simulink model "CONTROL_SYSTEM_V3_k"  (R2024a)
settings: Solver=ode1  StartTime=0.0  StopTime=inf  FixedStep=0.01  RelTol=1e-5
values from neighbouring files (symbols this model uses):
  Beta1 = 3*Omega_o    (= 15)    [CONTROL_SYSTEM_VAR.m]
  Beta2 = 3*(Omega_o^2)    (= 75)    [CONTROL_SYSTEM_VAR.m]
  Beta3 = (Omega_o^3)    (= 125)    [CONTROL_SYSTEM_VAR.m]
  Desire_Max = 255    [CONTROL_SYSTEM_VAR.m]
  Desire_Min = 0    [CONTROL_SYSTEM_VAR.m]
  Direction_Pin = 1    [CONTROL_SYSTEM_VAR.m]
  EN_Pin = 0    [CONTROL_SYSTEM_VAR.m]
  J_aet = 0.0035    [CONTROL_SYSTEM_VAR.m]
  Kd = 2    [CONTROL_SYSTEM_VAR.m]
  Ki = 4    [CONTROL_SYSTEM_VAR.m]
  Kn = 0.1    [CONTROL_SYSTEM_VAR.m]
  Kp = 1.4    [CONTROL_SYSTEM_VAR.m]
  omga_c = 10    [CONTROL_SYSTEM_VAR.m]
  roa = 0.24    [CONTROL_SYSTEM_VAR.m]
undefined symbols (not defined in the file or in its folder): sigbuilder_block
libraries: arduinolib x30, simulink_extras x14, simulink x5, slpidlib x4, spsOnDelayLib x2, slctrl_autotuning x2, slctrl_adaptive x1
(part 2 of 4)

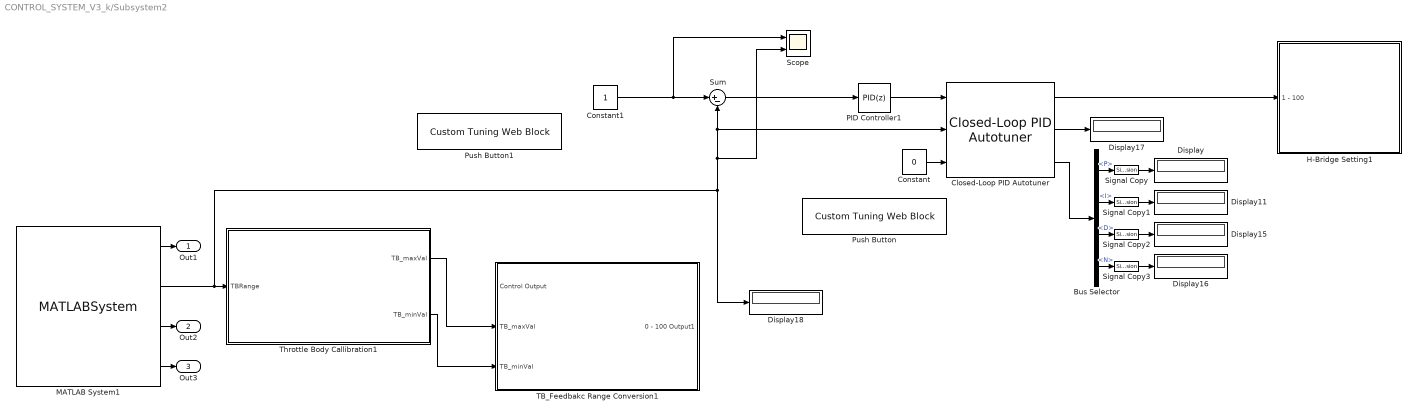
== system CONTROL_SYSTEM_V3_k/Subsystem2 ==
  Bus Selector : BusSelector  OutputSignals=P,I,D,N
  Closed-Loop PID Autotuner : slctrl_autotuning/Closed-Loop PID Autotuner  PIDType=PID  PIDForm=Parallel  TimeDomain=discrete-time  DiscreteTs=0.1  TuningTs=0.2  UseTuningTs=off  IntegratorFormula=Forward Euler  FilterFormula=Forward Euler  ContinuousTs=-1  Bandwidth=1  UseExternalWC=off  TargetPM=60  UseExternalPM=off  UseExternalAchievedPM=off  ExperimentMode=Superposition  PlantType=Stable  PlantSign=Positive  AmpSine=1  UseExternalAmpSine=off  UseExternalFRD=off  UseExternalU0=off  UseCompanion=off  NotDeployTuningModule=off  UsePLCCoder=off  OutputMode=control action + perturbation  BlockDataType=double  UseConnectedPID=on  blockpath=[]  tunedP=0  tunedI=0  tunedD=0  tunedN=100  tunedPM=0  EstimationWindowSize=3  UseExternalTuningParams=off  SingleMultiRateVariant=SingleSamplingRate  NumEstimationPeriods=4  NumSettlingPeriods=2  NumOfPRBSPeriod=1  PRBSSignalOrder=12  ExperimentModeVariant=VariantSuperimposed  OutputChoice=VariantCandD
      settings: LibrarySourceBlock=slctrlblks/Autotuning/Closed-Loop PID Autotuner
  Constant : Constant  Value=0
  Constant1 : Constant
  Display{,11,15..18} (6 alike) : Display
  H-Bridge Setting1 : Subsystem
      mask Display: image('H-Bridge.JPG');
  MATLAB System1 : MATLABSystem  System=ADS1115_Vread  SetGain=int16( 16 )  SampleTime=-1
      mask Type: ADS1115_Vread
      mask Display:
      | color('white');plot([100,100,100,100]*1,[100,100,100,100]*1);plot([100,100,100,100]*0,[100,100,100,100]*0);color('blue');text(38, 92, 'IO Device Builder','horizontalAlignment', 'right');
      | color('black');text(52,50,' ADS1115_Vread','horizontalAlignment','center');
      | port_label('output',1,'V0');port_label('output',2,'V1');port_label('output',3,'V2');port_label('output',4,'V3');
  PID Controller1 : slpidlib/PID Controller  Controller=PID  Form=Parallel  TimeDomain=Discrete-time  UseExternalTs=off  SampleTime=-1  IntegratorMethod=Forward Euler  FilterMethod=Forward Euler  ControllerParametersSource=internal  P=0  I=185.8371  UseKiTs=off  D=87.2762  UseExternalDerivativeSource=off  N=100  UseFilter=on  TunerSelectOption=Transfer Function Based (PID Tuner App)  InitialConditionSource=internal  InitialConditionForIntegrator=0  InitialConditionForFilter=0  DifferentiatorICPrevScaledInput=0  ExternalReset=none  TrackingMode=off  Kt=1  LimitOutput=off  SatLimitsSource=internal  UpperSaturationLimit=inf  LowerSaturationLimit=-inf  LinearizeAsGain=on  AntiWindupMode=none  Kb=1  LimitIntegrator=off  UpperIntegratorSaturationLimit=inf  LowerIntegratorSaturationLimit=-inf  POutMin=[]  POutMax=[]  IOutMin=[]  IOutMax=[]  DOutMin=[]  DOutMax=[]  NOutMin=[]  NOutMax=[]  SumOutMin=[]  SumOutMax=[]  SaturationOutMin=[]  SaturationOutMax=[]  PParamMin=[]  PParamMax=[]  IParamMin=[]  IParamMax=[]  DParamMin=[]  DParamMax=[]  NParamMin=[]  NParamMax=[]  KbParamMin=[]  KbParamMax=[]  KtParamMin=[]  KtParamMax=[]  KbOutMin=[]  KbOutMax=[]  KtOutMin=[]  KtOutMax=[]  IntegratorOutMin=[]  IntegratorOutMax=[]  FilterOutMin=[]  FilterOutMax=[]  SumI1OutMin=[]  SumI1OutMax=[]  SumI2OutMin=[]  SumI2OutMax=[]  SumI3OutMin=[]  SumI3OutMax=[]  SumI4OutMin=[]  SumI4OutMax=[]  SumDOutMin=[]  SumDOutMax=[]  DifferentiatorOutMin=[]  DifferentiatorOutMax=[]  FilterDiffOutCoefMin=[]  FilterDiffOutCoefMax=[]  ReciprocalOutMin=[]  ReciprocalOutMax=[]  SumDenOutMin=[]  SumDenOutMax=[]  SumNumOutMin=[]  SumNumOutMax=[]  DivideOutMin=[]  DivideOutMax=[]  UdiffTsProdOutMin=[]  UdiffTsProdOutMax=[]  NTsProdOutMin=[]  NTsProdOutMax=[]  UintegralTsProdOutMin=[]  UintegralTsProdOutMax=[]  UngainTsProdOutMin=[]  UngainTsProdOutMax=[]  ClampingZeroOutDataTypeStr=Inherit: Inherit via back propagation  ClampingZeroOutMin=[]  ClampingZeroOutMax=[]  FilterDenConstantOutDataTypeStr=Inherit: Inherit via back propagation  FilterDenConstantOutMin=[]  FilterDenConstantOutMax=[]  PCopyOutDataTypeStr=Inherit: Inherit via back propagation  PCopyOutMin=[]  PCopyOutMax=[]  NCopyOutDataTypeStr=Inherit: Inherit via back propagation  NCopyOutMin=[]  NCopyOutMax=[]  IntegratorContinuousStateAttributes=''  IntegratorStateMustResolveToSignalObject=off  IntegratorRTWStateStorageClass=Auto  FilterContinuousStateAttributes=''  FilterStateMustResolveToSignalObject=off  FilterRTWStateStorageClass=Auto  ParallelPVariant=InternalParameters  IdealPVariant=Disabled  IVariant=InternalParameters  DVariant=InternalParameters  IntegratorVariant=Discrete  SatVariant=Disabled  AWVariant=Passthrough  PCopyVariant=Disabled  TRVariant=Disabled  FdbkBlocksVariant=Forward  IdealPFdbkVariant=Disabled  SatFdbkVariant=Disabled  DerivativeFilterVariant=ForwardEulerFilter  NVariant=InternalParameters  NCopyVariant=Disabled  FilterICVariant=InternalICsFilter  IntegratorICVariant=InternalICs  ExternalResetVariant=Disabled  TRSumVariant=Passthrough  SumFdbkVariant=Disabled  SumVariant=Sum_PID  TsampFilterVariant=InternalTs  TsampNgainVariant=Passthrough  TsampIntegralVariant=Disabled_SignalSpec  ExternalSaturationOutDataTypeStr=Inherit: Same as second input  DerivativeSourceVariant=ErrorSignal
  Push Button : CustomTuningWebBlock  LabelPosition=Hide  ShowInitialText=on  Configuration="{\"components\":[{\"name\":\"BackgroundImageComponent\",\"settings\":{\"image\":{\"size\":[0,0],\"src\":\"default\",\"srcOrientation\":\"horizontal\"},\"position\":[0,0,1,1],\"scaleMode\":\"0\"}},{\"name\":\"ButtonStateComponent\",\"settings\":{\"buttonType\":\"latch\",\"clickFcn\":\"\",\"image\":{\"size\":[180,45],\"srcOrientation\":\"Right\"},\"latched\":false,\"offValue\":null,\"onValue\":\"1\",\"position\":[0,0,1,1],\"pressDelay\":\"500\",\"pressFcn\":\"\",\"repeatInterval\":\"0\",\"states\":[{\"horizontalAlignment\":\"center\",\"image\":{\"position\":[0.04444444444444445,0.005555555555555536,0.9888888888888889,0.9111111111111111],\"size\":[0.9888888888888889,0.9111111111111111],\"src\":\"data:image\\/svg+xml;base64,PHN2ZyB4bWxucz0iaHR0cDovL3d3dy53My5vcmcvMjAwMC9zdmciIHhtbG5zOnhsaW5rPSJodHRwOi8vd3d3LnczLm9yZy8xOTk5L3hsaW5rIiB2aWV3Qm94PSIwIDAgMTc3LjI1IDQwLjg4Ij48ZGVmcz48c3R5bGU+LmNscy0xe2ZpbGw6dXJsKCNyYWRpYWwtZ3JhZGllbnQpO30uY2xzLTJ7ZmlsbDp1cmwoI2xpbmVhci1ncmFkaWVudCk7fS5jbHMtM3tmaWxsOnVybCgjbGluZWFyLWdyYWRpZW50LTIpO308L3N0eWxlPjxyYWRpYWxHcmFkaWVudCBpZD0icmFkaWFsLWdyYWRpZW50IiBjeD0iOTAuMDkiIGN5PSIyMi42NiIgcj0i ...(+2212 chars)\",\"srcOrientation\":\"Right\"},\"label\":{\"color\":[1,1,0.78,1],\"icon\":{\"size\":[0.1,0.375],\"src\":\"data:image\\/svg+xml;base64,PHN2ZyBpZD0iT2ZmIiB4bWxucz0iaHR0cDovL3d3dy53My5vcmcvMjAwMC9zdmciIHhtbG5zOnhsaW5rPSJodHRwOi8vd3d3LnczLm9yZy8xOTk5L3hsaW5rIiB2aWV3Qm94PSIwIDAgNTAgNTAiPjxkZWZzPjxzdHlsZT4uY2xzLTF7ZmlsbDojN2Y4MDgwO3N0cm9rZTojMjcyNjI2O3N0cm9rZS1taXRlcmxpbWl0OjEwO3N0cm9rZS13aWR0aDozcHg7fS5jbHMtMntmaWxsOnVybCgjbGluZWFyLWdyYWRpZW50KTt9PC9zdHlsZT48bGluZWFyR3JhZGllbnQgaWQ9ImxpbmVhci1ncmFkaWVudCIgeDE9IjI1IiB5MT0iOSIgeDI9IjI1IiB5Mj0iMzciIGdyYWRpZW50VW5pdHM9InVzZXJTcGFjZU9uVXNlIj48c3RvcCBvZmZzZXQ9IjAiIHN0b3AtY29sb3I9IiNmZmYiIHN0b3Atb3BhY2l0eT0iMC43NSIvPjxzdG9wIG9mZnNldD0iMSIgc3RvcC1jb2xvcj0iI2ZmZiIgc3RvcC1vcGFjaXR5PSIwIi8+PC9saW5lYXJHcmFkaWVudD48L2RlZnM+PGNpcmNsZSBjbGFzcz0iY2xzLTEiIGN4PSIyNSIgY3k9IjI1IiByPSIyMCIvPjxjaXJjbGUgY2xhc3M9ImNscy0yIiBjeD0iMjUiIGN5PSIyMyIgcj0iMTQiLz48L3N2Zz4=\",\"srcOrientation\":\"Right\"},\"iconPlacement\":\"left\",\"opacity\":1,\"show\":true,\"text\":{\"content\":\"Button\",\"font\":\"Helvetica\",\"fontSize\":14}},\"labelOffset\":[0,0],\"verticalAlignment\":\"middle\"},{\"horizontalAlignment\":\"center\",\"image\":{\"position\":[0.04444444444444445,0.005555555555555536,0.9888888888888889,0.9111111111111111],\"size\":[0.9888888888888889,0.9111111111111111],\"src\":\"data:image\\/svg+xml;base64,PHN2ZyB4bWxucz0iaHR0cDovL3d3dy53My5vcmcvMjAwMC9zdmciIHhtbG5zOnhsaW5rPSJodHRwOi8vd3d3LnczLm9yZy8xOTk5L3hsaW5rIiB2aWV3Qm94PSIwIDAgMTc3LjI1IDQwLjg4Ij48ZGVmcz48c3R5bGU+LmNscy0xe2ZpbGw6dXJsKCNyYWRpYWwtZ3JhZGllbnQpO30uY2xzLTJ7ZmlsbDp1cmwoI2xpbmVhci1ncmFkaWVudCk7fS5jbHMtM3tmaWxsOnVybCgjbGluZWFyLWdyYWRpZW50LTIpO308L3N0eWxlPjxyYWRpYWxHcmFkaWVudCBpZD0icmFkaWFsLWdyYWRpZW50IiBjeD0iOTAuMDkiIGN5PSIyMi42NiIgcj0i ...(+2216 chars)\",\"srcOrientation\":\"Right\"},\"label\":{\"color\":[1,1,0.78,1],\"icon\":{\"size\":[0.1,0.375],\"src\":\"data:image\\/svg+xml;base64,PHN2ZyB4bWxucz0iaHR0cDovL3d3dy53My5vcmcvMjAwMC9zdmciIHhtbG5zOnhsaW5rPSJodHRwOi8vd3d3LnczLm9yZy8xOTk5L3hsaW5rIiB2aWV3Qm94PSIwIDAgNTAgNTAiPjxkZWZzPjxzdHlsZT4uY2xzLTF7ZmlsbDojNmFiZDQ1O3N0cm9rZTojMjcyNjI2O3N0cm9rZS1taXRlcmxpbWl0OjEwO3N0cm9rZS13aWR0aDozcHg7fS5jbHMtMntmaWxsOnVybCgjbGluZWFyLWdyYWRpZW50KTt9PC9zdHlsZT48bGluZWFyR3JhZGllbnQgaWQ9ImxpbmVhci1ncmFkaWVudCIgeDE9IjI1IiB5MT0iOSIgeDI9IjI1IiB5Mj0iMzciIGdyYWRpZW50VW5pdHM9InVzZXJTcGFjZU9uVXNlIj48c3RvcCBvZmZzZXQ9IjAiIHN0b3AtY29sb3I9IiNmZmYiIHN0b3Atb3BhY2l0eT0iMC43NSIvPjxzdG9wIG9mZnNldD0iMSIgc3RvcC1jb2xvcj0iI2ZmZiIgc3RvcC1vcGFjaXR5PSIwIi8+PC9saW5lYXJHcmFkaWVudD48L2RlZnM+PGcgaWQ9Ik9uIj48Y2lyY2xlIGNsYXNzPSJjbHMtMSIgY3g9IjI1IiBjeT0iMjUiIHI9IjIwIi8+PGNpcmNsZSBjbGFzcz0iY2xzLTIiIGN4PSIyNSIgY3k9IjIzIiByPSIxNCIvPjwvZz48L3N2Zz4=\",\"srcOrientation\":\"Right\"},\"iconPlacement\":\"left\",\"opacity\":1,\"show\":true,\"text\":{\"content\":\"Button\",\"font\":\"Helvetica\",\"fontSize\":14}},\"labelOffset\":[0.025,0],\"verticalAlignment\":\"middle\"},{\"horizontalAlignment\":\"center\",\"image\":{\"position\":[0.04444444444444445,0.005555555555555536,0.9888888888888889,0.9111111111111111],\"size\":[0.9888888888888889,0.9111111111111111],\"src\":\"data:image\\/svg+xml;base64,PHN2ZyB4bWxucz0iaHR0cDovL3d3dy53My5vcmcvMjAwMC9zdmciIHhtbG5zOnhsaW5rPSJodHRwOi8vd3d3LnczLm9yZy8xOTk5L3hsaW5rIiB2aWV3Qm94PSIwIDAgMTc3LjI1IDQwLjg4Ij48ZGVmcz48c3R5bGU+LmNscy0xe2ZpbGw6dXJsKCNyYWRpYWwtZ3JhZGllbnQpO30uY2xzLTJ7ZmlsbDp1cmwoI2xpbmVhci1ncmFkaWVudCk7fS5jbHMtM3tmaWxsOnVybCgjbGluZWFyLWdyYWRpZW50LTIpO308L3N0eWxlPjxyYWRpYWxHcmFkaWVudCBpZD0icmFkaWFsLWdyYWRpZW50IiBjeD0iOTAuMDkiIGN5PSIyMi42NiIgcj0i ...(+2212 chars)\",\"srcOrientation\":\"Right\"},\"label\":{\"color\":[1,1,0.78,1],\"icon\":{\"size\":[0.1,0.375],\"src\":\"data:image\\/svg+xml;base64,PHN2ZyB4bWxucz0iaHR0cDovL3d3dy53My5vcmcvMjAwMC9zdmciIHhtbG5zOnhsaW5rPSJodHRwOi8vd3d3LnczLm9yZy8xOTk5L3hsaW5rIiB2aWV3Qm94PSIwIDAgNTAgNTAiPjxkZWZzPjxzdHlsZT4uY2xzLTF7ZmlsbDojNmFiZDQ1O3N0cm9rZTojMjcyNjI2O3N0cm9rZS1taXRlcmxpbWl0OjEwO3N0cm9rZS13aWR0aDozcHg7fS5jbHMtMntmaWxsOnVybCgjbGluZWFyLWdyYWRpZW50KTt9PC9zdHlsZT48bGluZWFyR3JhZGllbnQgaWQ9ImxpbmVhci1ncmFkaWVudCIgeDE9IjI1IiB5MT0iOSIgeDI9IjI1IiB5Mj0iMzciIGdyYWRpZW50VW5pdHM9InVzZXJTcGFjZU9uVXNlIj48c3RvcCBvZmZzZXQ9IjAiIHN0b3AtY29sb3I9IiNmZmYiIHN0b3Atb3BhY2l0eT0iMC43NSIvPjxzdG9wIG9mZnNldD0iMSIgc3RvcC1jb2xvcj0iI2ZmZiIgc3RvcC1vcGFjaXR5PSIwIi8+PC9saW5lYXJHcmFkaWVudD48L2RlZnM+PGcgaWQ9Ik9uIj48Y2lyY2xlIGNsYXNzPSJjbHMtMSIgY3g9IjI1IiBjeT0iMjUiIHI9IjIwIi8+PGNpcmNsZSBjbGFzcz0iY2xzLTIiIGN4PSIyNSIgY3k9IjIzIiByPSIxNCIvPjwvZz48L3N2Zz4=\",\"srcOrientation\":\"Right\"},\"iconPlacement\":\"left\",\"opacity\":1,\"show\":true,\"text\":{\"content\":\"Button\",\"font\":\"Helvetica\",\"fontSize\":14}},\"labelOffset\":[0,0],\"verticalAlignment\":\"middle\"},{\"horizontalAlignment\":\"center\",\"image\":{\"position\":[0.04444444444444445,0.005555555555555536,0.9888888888888889,0.9111111111111111],\"size\":[0.9888888888888889,0.9111111111111111],\"src\":\"data:image\\/svg+xml;base64,PHN2ZyB4bWxucz0iaHR0cDovL3d3dy53My5vcmcvMjAwMC9zdmciIHhtbG5zOnhsaW5rPSJodHRwOi8vd3d3LnczLm9yZy8xOTk5L3hsaW5rIiB2aWV3Qm94PSIwIDAgMTc3LjI1IDQwLjg4Ij48ZGVmcz48c3R5bGU+LmNscy0xe2ZpbGw6dXJsKCNyYWRpYWwtZ3JhZGllbnQpO30uY2xzLTJ7ZmlsbDp1cmwoI2xpbmVhci1ncmFkaWVudCk7fS5jbHMtM3tmaWxsOnVybCgjbGluZWFyLWdyYWRpZW50LTIpO308L3N0eWxlPjxyYWRpYWxHcmFkaWVudCBpZD0icmFkaWFsLWdyYWRpZW50IiBjeD0iOTAuMDkiIGN5PSIyMi42NiIgcj0i ...(+2216 chars)\",\"srcOrientation\":\"Right\"},\"label\":{\"color\":[1,1,0.78,1],\"icon\":{\"size\":[0.1,0.375],\"src\":\"data:image\\/svg+xml;base64,PHN2ZyBpZD0iT2ZmIiB4bWxucz0iaHR0cDovL3d3dy53My5vcmcvMjAwMC9zdmciIHhtbG5zOnhsaW5rPSJodHRwOi8vd3d3LnczLm9yZy8xOTk5L3hsaW5rIiB2aWV3Qm94PSIwIDAgNTAgNTAiPjxkZWZzPjxzdHlsZT4uY2xzLTF7ZmlsbDojN2Y4MDgwO3N0cm9rZTojMjcyNjI2O3N0cm9rZS1taXRlcmxpbWl0OjEwO3N0cm9rZS13aWR0aDozcHg7fS5jbHMtMntmaWxsOnVybCgjbGluZWFyLWdyYWRpZW50KTt9PC9zdHlsZT48bGluZWFyR3JhZGllbnQgaWQ9ImxpbmVhci1ncmFkaWVudCIgeDE9IjI1IiB5MT0iOSIgeDI9IjI1IiB5Mj0iMzciIGdyYWRpZW50VW5pdHM9InVzZXJTcGFjZU9uVXNlIj48c3RvcCBvZmZzZXQ9IjAiIHN0b3AtY29sb3I9IiNmZmYiIHN0b3Atb3BhY2l0eT0iMC43NSIvPjxzdG9wIG9mZnNldD0iMSIgc3RvcC1jb2xvcj0iI2ZmZiIgc3RvcC1vcGFjaXR5PSIwIi8+PC9saW5lYXJHcmFkaWVudD48L2RlZnM+PGNpcmNsZSBjbGFzcz0iY2xzLTEiIGN4PSIyNSIgY3k9IjI1IiByPSIyMCIvPjxjaXJjbGUgY2xhc3M9ImNscy0yIiBjeD0iMjUiIGN5PSIyMyIgcj0iMTQiLz48L3N2Zz4=\",\"srcOrientation\":\"Right\"},\"iconPlacement\":\"left\",\"opacity\":1,\"show\":true,\"text\":{\"content\":\"Button\",\"font\":\"Helvetica\",\"fontSize\":14}},\"labelOffset\":[0.025,0],\"verticalAlignment\":\"middle\"}]}},{\"name\":\"ForegroundImageComponent\",\"settings\":{\"image\":{\"size\":[0,0],\"src\":\"default\",\"srcOrientation\":\"horizontal\"},\"isForeground\":1,\"position\":[0,0,1,1],\"scaleMode\":\"0\"}}],\"settings\":{\"BindingType\":\"param\",\"aspectRatio\":3.7777777777777777,\"backgroundColor\":[0,0,0,\"1\"],\"backgroundOffset\":0,\"backgroundOpacity\":1,\"fixedAspectRatio\":\"on\",\"foregroundColor\":[252,252,196],\"showBackgroundColor\":false,\"variant\":\"push\",\"version\":\"R2023a\"},\"type\":\"Button\"}"
  Push Button1 : CustomTuningWebBlock  LabelPosition=Hide  ShowInitialText=on  Configuration="{\"components\":[{\"name\":\"BackgroundImageComponent\",\"settings\":{\"image\":{\"size\":[0,0],\"src\":\"default\",\"srcOrientation\":\"horizontal\"},\"position\":[0,0,1,1],\"scaleMode\":\"0\"}},{\"name\":\"ButtonStateComponent\",\"settings\":{\"buttonType\":\"latch\",\"clickFcn\":\"\",\"image\":{\"size\":[180,45],\"srcOrientation\":\"Right\"},\"latched\":true,\"offValue\":0,\"onValue\":\"1\",\"position\":[0,0,1,1],\"pressDelay\":\"500\",\"pressFcn\":\"\",\"repeatInterval\":\"0\",\"states\":[{\"horizontalAlignment\":\"center\",\"image\":{\"position\":[0.04444444444444445,0.005555555555555536,0.9888888888888889,0.9111111111111111],\"size\":[0.9888888888888889,0.9111111111111111],\"src\":\"data:image\\/svg+xml;base64,PHN2ZyB4bWxucz0iaHR0cDovL3d3dy53My5vcmcvMjAwMC9zdmciIHhtbG5zOnhsaW5rPSJodHRwOi8vd3d3LnczLm9yZy8xOTk5L3hsaW5rIiB2aWV3Qm94PSIwIDAgMTc3LjI1IDQwLjg4Ij48ZGVmcz48c3R5bGU+LmNscy0xe2ZpbGw6dXJsKCNyYWRpYWwtZ3JhZGllbnQpO30uY2xzLTJ7ZmlsbDp1cmwoI2xpbmVhci1ncmFkaWVudCk7fS5jbHMtM3tmaWxsOnVybCgjbGluZWFyLWdyYWRpZW50LTIpO308L3N0eWxlPjxyYWRpYWxHcmFkaWVudCBpZD0icmFkaWFsLWdyYWRpZW50IiBjeD0iOTAuMDkiIGN5PSIyMi42NiIgcj0i ...(+2212 chars)\",\"srcOrientation\":\"Right\"},\"label\":{\"color\":[1,1,0.78,1],\"icon\":{\"size\":[0.1,0.375],\"src\":\"data:image\\/svg+xml;base64,PHN2ZyBpZD0iT2ZmIiB4bWxucz0iaHR0cDovL3d3dy53My5vcmcvMjAwMC9zdmciIHhtbG5zOnhsaW5rPSJodHRwOi8vd3d3LnczLm9yZy8xOTk5L3hsaW5rIiB2aWV3Qm94PSIwIDAgNTAgNTAiPjxkZWZzPjxzdHlsZT4uY2xzLTF7ZmlsbDojN2Y4MDgwO3N0cm9rZTojMjcyNjI2O3N0cm9rZS1taXRlcmxpbWl0OjEwO3N0cm9rZS13aWR0aDozcHg7fS5jbHMtMntmaWxsOnVybCgjbGluZWFyLWdyYWRpZW50KTt9PC9zdHlsZT48bGluZWFyR3JhZGllbnQgaWQ9ImxpbmVhci1ncmFkaWVudCIgeDE9IjI1IiB5MT0iOSIgeDI9IjI1IiB5Mj0iMzciIGdyYWRpZW50VW5pdHM9InVzZXJTcGFjZU9uVXNlIj48c3RvcCBvZmZzZXQ9IjAiIHN0b3AtY29sb3I9IiNmZmYiIHN0b3Atb3BhY2l0eT0iMC43NSIvPjxzdG9wIG9mZnNldD0iMSIgc3RvcC1jb2xvcj0iI2ZmZiIgc3RvcC1vcGFjaXR5PSIwIi8+PC9saW5lYXJHcmFkaWVudD48L2RlZnM+PGNpcmNsZSBjbGFzcz0iY2xzLTEiIGN4PSIyNSIgY3k9IjI1IiByPSIyMCIvPjxjaXJjbGUgY2xhc3M9ImNscy0yIiBjeD0iMjUiIGN5PSIyMyIgcj0iMTQiLz48L3N2Zz4=\",\"srcOrientation\":\"Right\"},\"iconPlacement\":\"left\",\"opacity\":1,\"show\":true,\"text\":{\"content\":\"Button\",\"font\":\"Helvetica\",\"fontSize\":14}},\"labelOffset\":[0,0],\"verticalAlignment\":\"middle\"},{\"horizontalAlignment\":\"center\",\"image\":{\"position\":[0.04444444444444445,0.005555555555555536,0.9888888888888889,0.9111111111111111],\"size\":[0.9888888888888889,0.9111111111111111],\"src\":\"data:image\\/svg+xml;base64,PHN2ZyB4bWxucz0iaHR0cDovL3d3dy53My5vcmcvMjAwMC9zdmciIHhtbG5zOnhsaW5rPSJodHRwOi8vd3d3LnczLm9yZy8xOTk5L3hsaW5rIiB2aWV3Qm94PSIwIDAgMTc3LjI1IDQwLjg4Ij48ZGVmcz48c3R5bGU+LmNscy0xe2ZpbGw6dXJsKCNyYWRpYWwtZ3JhZGllbnQpO30uY2xzLTJ7ZmlsbDp1cmwoI2xpbmVhci1ncmFkaWVudCk7fS5jbHMtM3tmaWxsOnVybCgjbGluZWFyLWdyYWRpZW50LTIpO308L3N0eWxlPjxyYWRpYWxHcmFkaWVudCBpZD0icmFkaWFsLWdyYWRpZW50IiBjeD0iOTAuMDkiIGN5PSIyMi42NiIgcj0i ...(+2216 chars)\",\"srcOrientation\":\"Right\"},\"label\":{\"color\":[1,1,0.78,1],\"icon\":{\"size\":[0.1,0.375],\"src\":\"data:image\\/svg+xml;base64,PHN2ZyB4bWxucz0iaHR0cDovL3d3dy53My5vcmcvMjAwMC9zdmciIHhtbG5zOnhsaW5rPSJodHRwOi8vd3d3LnczLm9yZy8xOTk5L3hsaW5rIiB2aWV3Qm94PSIwIDAgNTAgNTAiPjxkZWZzPjxzdHlsZT4uY2xzLTF7ZmlsbDojNmFiZDQ1O3N0cm9rZTojMjcyNjI2O3N0cm9rZS1taXRlcmxpbWl0OjEwO3N0cm9rZS13aWR0aDozcHg7fS5jbHMtMntmaWxsOnVybCgjbGluZWFyLWdyYWRpZW50KTt9PC9zdHlsZT48bGluZWFyR3JhZGllbnQgaWQ9ImxpbmVhci1ncmFkaWVudCIgeDE9IjI1IiB5MT0iOSIgeDI9IjI1IiB5Mj0iMzciIGdyYWRpZW50VW5pdHM9InVzZXJTcGFjZU9uVXNlIj48c3RvcCBvZmZzZXQ9IjAiIHN0b3AtY29sb3I9IiNmZmYiIHN0b3Atb3BhY2l0eT0iMC43NSIvPjxzdG9wIG9mZnNldD0iMSIgc3RvcC1jb2xvcj0iI2ZmZiIgc3RvcC1vcGFjaXR5PSIwIi8+PC9saW5lYXJHcmFkaWVudD48L2RlZnM+PGcgaWQ9Ik9uIj48Y2lyY2xlIGNsYXNzPSJjbHMtMSIgY3g9IjI1IiBjeT0iMjUiIHI9IjIwIi8+PGNpcmNsZSBjbGFzcz0iY2xzLTIiIGN4PSIyNSIgY3k9IjIzIiByPSIxNCIvPjwvZz48L3N2Zz4=\",\"srcOrientation\":\"Right\"},\"iconPlacement\":\"left\",\"opacity\":1,\"show\":true,\"text\":{\"content\":\"Button\",\"font\":\"Helvetica\",\"fontSize\":14}},\"labelOffset\":[0.025,0],\"verticalAlignment\":\"middle\"},{\"horizontalAlignment\":\"center\",\"image\":{\"position\":[0.04444444444444445,0.005555555555555536,0.9888888888888889,0.9111111111111111],\"size\":[0.9888888888888889,0.9111111111111111],\"src\":\"data:image\\/svg+xml;base64,PHN2ZyB4bWxucz0iaHR0cDovL3d3dy53My5vcmcvMjAwMC9zdmciIHhtbG5zOnhsaW5rPSJodHRwOi8vd3d3LnczLm9yZy8xOTk5L3hsaW5rIiB2aWV3Qm94PSIwIDAgMTc3LjI1IDQwLjg4Ij48ZGVmcz48c3R5bGU+LmNscy0xe2ZpbGw6dXJsKCNyYWRpYWwtZ3JhZGllbnQpO30uY2xzLTJ7ZmlsbDp1cmwoI2xpbmVhci1ncmFkaWVudCk7fS5jbHMtM3tmaWxsOnVybCgjbGluZWFyLWdyYWRpZW50LTIpO308L3N0eWxlPjxyYWRpYWxHcmFkaWVudCBpZD0icmFkaWFsLWdyYWRpZW50IiBjeD0iOTAuMDkiIGN5PSIyMi42NiIgcj0i ...(+2212 chars)\",\"srcOrientation\":\"Right\"},\"label\":{\"color\":[1,1,0.78,1],\"icon\":{\"size\":[0.1,0.375],\"src\":\"data:image\\/svg+xml;base64,PHN2ZyB4bWxucz0iaHR0cDovL3d3dy53My5vcmcvMjAwMC9zdmciIHhtbG5zOnhsaW5rPSJodHRwOi8vd3d3LnczLm9yZy8xOTk5L3hsaW5rIiB2aWV3Qm94PSIwIDAgNTAgNTAiPjxkZWZzPjxzdHlsZT4uY2xzLTF7ZmlsbDojNmFiZDQ1O3N0cm9rZTojMjcyNjI2O3N0cm9rZS1taXRlcmxpbWl0OjEwO3N0cm9rZS13aWR0aDozcHg7fS5jbHMtMntmaWxsOnVybCgjbGluZWFyLWdyYWRpZW50KTt9PC9zdHlsZT48bGluZWFyR3JhZGllbnQgaWQ9ImxpbmVhci1ncmFkaWVudCIgeDE9IjI1IiB5MT0iOSIgeDI9IjI1IiB5Mj0iMzciIGdyYWRpZW50VW5pdHM9InVzZXJTcGFjZU9uVXNlIj48c3RvcCBvZmZzZXQ9IjAiIHN0b3AtY29sb3I9IiNmZmYiIHN0b3Atb3BhY2l0eT0iMC43NSIvPjxzdG9wIG9mZnNldD0iMSIgc3RvcC1jb2xvcj0iI2ZmZiIgc3RvcC1vcGFjaXR5PSIwIi8+PC9saW5lYXJHcmFkaWVudD48L2RlZnM+PGcgaWQ9Ik9uIj48Y2lyY2xlIGNsYXNzPSJjbHMtMSIgY3g9IjI1IiBjeT0iMjUiIHI9IjIwIi8+PGNpcmNsZSBjbGFzcz0iY2xzLTIiIGN4PSIyNSIgY3k9IjIzIiByPSIxNCIvPjwvZz48L3N2Zz4=\",\"srcOrientation\":\"Right\"},\"iconPlacement\":\"left\",\"opacity\":1,\"show\":true,\"text\":{\"content\":\"Button\",\"font\":\"Helvetica\",\"fontSize\":14}},\"labelOffset\":[0,0],\"verticalAlignment\":\"middle\"},{\"horizontalAlignment\":\"center\",\"image\":{\"position\":[0.04444444444444445,0.005555555555555536,0.9888888888888889,0.9111111111111111],\"size\":[0.9888888888888889,0.9111111111111111],\"src\":\"data:image\\/svg+xml;base64,PHN2ZyB4bWxucz0iaHR0cDovL3d3dy53My5vcmcvMjAwMC9zdmciIHhtbG5zOnhsaW5rPSJodHRwOi8vd3d3LnczLm9yZy8xOTk5L3hsaW5rIiB2aWV3Qm94PSIwIDAgMTc3LjI1IDQwLjg4Ij48ZGVmcz48c3R5bGU+LmNscy0xe2ZpbGw6dXJsKCNyYWRpYWwtZ3JhZGllbnQpO30uY2xzLTJ7ZmlsbDp1cmwoI2xpbmVhci1ncmFkaWVudCk7fS5jbHMtM3tmaWxsOnVybCgjbGluZWFyLWdyYWRpZW50LTIpO308L3N0eWxlPjxyYWRpYWxHcmFkaWVudCBpZD0icmFkaWFsLWdyYWRpZW50IiBjeD0iOTAuMDkiIGN5PSIyMi42NiIgcj0i ...(+2216 chars)\",\"srcOrientation\":\"Right\"},\"label\":{\"color\":[1,1,0.78,1],\"icon\":{\"size\":[0.1,0.375],\"src\":\"data:image\\/svg+xml;base64,PHN2ZyBpZD0iT2ZmIiB4bWxucz0iaHR0cDovL3d3dy53My5vcmcvMjAwMC9zdmciIHhtbG5zOnhsaW5rPSJodHRwOi8vd3d3LnczLm9yZy8xOTk5L3hsaW5rIiB2aWV3Qm94PSIwIDAgNTAgNTAiPjxkZWZzPjxzdHlsZT4uY2xzLTF7ZmlsbDojN2Y4MDgwO3N0cm9rZTojMjcyNjI2O3N0cm9rZS1taXRlcmxpbWl0OjEwO3N0cm9rZS13aWR0aDozcHg7fS5jbHMtMntmaWxsOnVybCgjbGluZWFyLWdyYWRpZW50KTt9PC9zdHlsZT48bGluZWFyR3JhZGllbnQgaWQ9ImxpbmVhci1ncmFkaWVudCIgeDE9IjI1IiB5MT0iOSIgeDI9IjI1IiB5Mj0iMzciIGdyYWRpZW50VW5pdHM9InVzZXJTcGFjZU9uVXNlIj48c3RvcCBvZmZzZXQ9IjAiIHN0b3AtY29sb3I9IiNmZmYiIHN0b3Atb3BhY2l0eT0iMC43NSIvPjxzdG9wIG9mZnNldD0iMSIgc3RvcC1jb2xvcj0iI2ZmZiIgc3RvcC1vcGFjaXR5PSIwIi8+PC9saW5lYXJHcmFkaWVudD48L2RlZnM+PGNpcmNsZSBjbGFzcz0iY2xzLTEiIGN4PSIyNSIgY3k9IjI1IiByPSIyMCIvPjxjaXJjbGUgY2xhc3M9ImNscy0yIiBjeD0iMjUiIGN5PSIyMyIgcj0iMTQiLz48L3N2Zz4=\",\"srcOrientation\":\"Right\"},\"iconPlacement\":\"left\",\"opacity\":1,\"show\":true,\"text\":{\"content\":\"Button\",\"font\":\"Helvetica\",\"fontSize\":14}},\"labelOffset\":[0.025,0],\"verticalAlignment\":\"middle\"}]}},{\"name\":\"ForegroundImageComponent\",\"settings\":{\"image\":{\"size\":[0,0],\"src\":\"default\",\"srcOrientation\":\"horizontal\"},\"isForeground\":1,\"position\":[0,0,1,1],\"scaleMode\":\"0\"}}],\"settings\":{\"BindingType\":\"param\",\"aspectRatio\":3.7777777777777777,\"backgroundColor\":[0,0,0,\"1\"],\"backgroundOffset\":0,\"backgroundOpacity\":1,\"fixedAspectRatio\":\"on\",\"foregroundColor\":[252,252,196],\"showBackgroundColor\":false,\"variant\":\"push\",\"version\":\"R2023a\"},\"type\":\"Button\"}"
  Scope : Scope  NumInputPorts=2
  Signal Copy{,1..3} (4 alike) : SignalConversion  OverrideOpt=off
  Sum : Sum  Inputs=|+-
  TB_Feedbakc Range Conversion1 : Subsystem
  Throttle Body Callibration1 : MATLAB Function  TreatAsAtomicUnit=on
  Out1 : Outport
  Out2 : Outport  Port=2
  Out3 : Outport  Port=3
  wires:
  Signal Copy/1 -> Display/1
  Closed-Loop PID Autotuner/1 -> H-Bridge Setting1/1(1 - 100)
  Bus Selector/3 -> Signal Copy2/1  "<D>"
  Constant/1 -> Closed-Loop PID Autotuner/3
  MATLAB System1/4 -> Out3/1
  Closed-Loop PID Autotuner/3 -> Bus Selector/1
  MATLAB System1/2 -> Scope/2, Closed-Loop PID Autotuner/2, Sum/2, Display18/1, Throttle Body Callibration1/1(TBRange)
  Closed-Loop PID Autotuner/2 -> Display17/1
  Signal Copy2/1 -> Display15/1
  Bus Selector/4 -> Signal Copy3/1  "<N>"
  Signal Copy1/1 -> Display11/1
  Bus Selector/2 -> Signal Copy1/1  "<I>"
  Bus Selector/1 -> Signal Copy/1  "<P>"
  Signal Copy3/1 -> Display16/1
  Constant1/1 -> Scope/1, Sum/1
  Throttle Body Callibration1/2(TB_minVal) -> TB_Feedbakc Range Conversion1/3(TB_minVal)
  Throttle Body Callibration1/1(TB_maxVal) -> TB_Feedbakc Range Conversion1/2(TB_maxVal)
  PID Controller1/1 -> Closed-Loop PID Autotuner/1
  Sum/1 -> PID Controller1/1
  MATLAB System1/1 -> Out1/1
  MATLAB System1/3 -> Out2/1

== system CONTROL_SYSTEM_V3_k/Subsystem4 ==
  TBRange : Inport
  Calibration_Input : Inport  Port=2
  PedalRange : Inport  Port=3
  Calibration_Input1 : Inport  Port=4
  Enable : EnablePort
  Pedal Calibration2 : MATLAB Function  TreatAsAtomicUnit=on
  Throttle Body Callibration1 : MATLAB Function  TreatAsAtomicUnit=on
  TB_maxVal : Outport
  TB_minVal : Outport  Port=2
  FP_maxVal : Outport  Port=3
  FP_minVal : Outport  Port=4
  wires:
  Calibration_Input1/1 -> Pedal Calibration2/2(Calibration_Input)
  TBRange/1 -> Throttle Body Callibration1/1(TBRange)
  Throttle Body Callibration1/2(TB_minVal) -> TB_minVal/1
  PedalRange/1 -> Pedal Calibration2/1(PedalRange)
  Pedal Calibration2/2(FP_minVal) -> FP_minVal/1
  Calibration_Input/1 -> Throttle Body Callibration1/2(Calibration_Input)
  Throttle Body Callibration1/1(TB_maxVal) -> TB_maxVal/1
  Pedal Calibration2/1(FP_maxVal) -> FP_maxVal/1

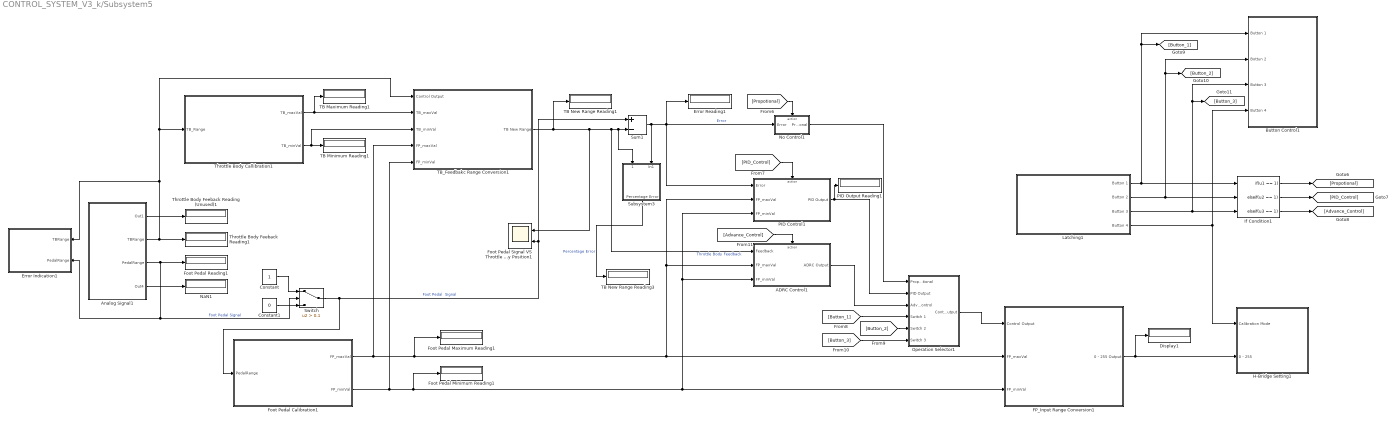
== system CONTROL_SYSTEM_V3_k/Subsystem5 ==
  ADRC Control1 : Subsystem
  Analog Signal1 : Subsystem
      mask Display: image('Capture.JPG');
  Button Control1 : Subsystem
  Constant : Constant
  Constant1 : Constant  Value=0
  Display1 : Display
      settings: Decimation=2
  Error Indication1 : Subsystem
      settings: PortSchema="{\"entries\":[{\"content\":{\"sides\":[{\"content\":{},\"type\":\"ConnectorPlacement.EquallySpacedRectSide\",\"uuid\":\"6bb27259-0fc4-412b-bd28-187413250838\"},{\"content\":{\"connectorIds\":[\"In1\",\"In2\"],\"side\":\"RIGHT\"},\"type\":\"ConnectorPlacement.EquallySpacedRectSide\",\"uuid\":\"b38a583a-7cdb-4b72-8a0e-445370b0f03f\"},{\"content\":{\"side\":\"TOP\"},\"type\":\"ConnectorPlacement.EquallySpacedRectSide\",\"uuid\":\"477ad40e-8e68-4653-afaf-50b4ab734c9d\"}]},\"type\":\"ConnectorPlacement.EquallySpacedConnector\",\"uuid\":\"474c0f68-6b48-44ee-b6ec-af4e49acdc40\"}],\"packageUris\":[\"http://schema.mathworks.com/mf0/Connector/R2020b\"],\"version\":\"1.0\"}"
  Error Reading1 : Display
      settings: Decimation=2
  FP_Input Range Conversion1 : Subsystem
  Foot Pedal Calibration1 : MATLAB Function  TreatAsAtomicUnit=on
  Foot Pedal Maximum Reading1 : Display
      settings: Decimation=2
  Foot Pedal Minimum Reading1 : Display
      settings: Decimation=2
  Foot Pedal Reading1 : Display
      settings: Decimation=2
  Foot Pedal Signal VS Throttle Body Position1 : Scope  NumInputPorts=2
  H-Bridge Setting1 : Subsystem
      mask Display: image('H-Bridge-removebg-preview.png');
  If Condition1 : If  NumInputs=3  IfExpression=u1 == 1  ElseIfExpressions=u2 == 1, u3 == 1  ShowElse=off
  Latching1 : Subsystem
  NaN1 : Display
      settings: Decimation=2
  No Control1 : Subsystem  TreatAsAtomicUnit=on
  Operation Selector1 : Subsystem
  PID Control1 : Subsystem
  PID Output Reading1 : Display
      settings: Decimation=2
  Subsystem3 : Subsystem
      settings: PortSchema="{\"entries\":[{\"content\":{\"sides\":[{\"content\":{},\"type\":\"ConnectorPlacement.EquallySpacedRectSide\",\"uuid\":\"06ab9b8c-dc11-4e78-9aea-2a49b899d383\"},{\"content\":{\"side\":\"RIGHT\"},\"type\":\"ConnectorPlacement.EquallySpacedRectSide\",\"uuid\":\"ea81575a-6f3e-44ea-98d6-a15110b05ea2\"},{\"content\":{\"connectorIds\":[\"In1\",\"In2\"],\"side\":\"TOP\"},\"type\":\"ConnectorPlacement.EquallySpacedRectSide\",\"uuid\":\"b4582e74-93d2-4cba-bd7b-a3215d2fef1c\"},{\"content\":{\"connectorIds\":[\"Out1\"],\"side\":\"BOTTOM\"},\"type\":\"ConnectorPlacement.EquallySpacedRectSide\",\"uuid\":\"d3012ec7-4a68-4cee-bd0d-e63c4f089545\"}]},\"type\":\"ConnectorPlacement.EquallySpacedConnector\",\"uuid\":\"85ff3d74-6a46-44e9-8a38-f9999c5d3ee8\"}],\"packageUris\":[\"http://schema.mathworks.com/mf0/Connector/R2020b\"],\"version\":\"1.0\"}"
  Sum1 : Sum  Inputs=+-
  Switch : Switch  Criteria=u2 > Threshold  Threshold=0.1  SaturateOnIntegerOverflow=off  InputSameDT=off
  TB Maximum Reading1 : Display
      settings: Decimation=2
  TB Minimum Reading1 : Display
      settings: Decimation=2
  TB New Range Reading1 : Display
      settings: Decimation=2
  TB New Range Reading3 : Display
      settings: Decimation=2
  TB_Feedbakc Range Conversion1 : Subsystem
  Throttle Body Callibration1 : MATLAB Function  TreatAsAtomicUnit=on
  Throttle Body Feeback Reading (Unused)1 : Display
      settings: Decimation=2
  Throttle Body Feeback Reading1 : Display
      settings: Decimation=2
  wires:
  Latching1/4(Button 4) -> H-Bridge Setting1/1(Calibration Mode), Button Control1/4(Button 4)
  TB_Feedbakc Range Conversion1/1(TB New Range) -> Foot Pedal Signal VS Throttle Body Position1/1, ADRC Control1/1(Feedback), Sum1/2, Subsystem3/1(Throttle Body Feedback), TB New Range Reading1/1  "Throttle Body Feedback"
  Switch/1 -> Foot Pedal Calibration1/1(PedalRange), Sum1/1, Foot Pedal Signal VS Throttle Body Position1/2  "Foot Pedal  Signal"
  Analog Signal1/4(Out4) -> NaN1/1
  If Condition1/3 -> [Advance_Control]
  Constant1/1 -> Switch/3
  FP_Input Range Conversion1/1(0 - 255 Output) -> H-Bridge Setting1/2(0 - 255), Display1/1
  Analog Signal1/3(PedalRange) -> Foot Pedal Reading1/1, Switch/2, Error Indication1/2(PedalRange)  "Foot Pedal Signal"
  Analog Signal1/2(TBRange) -> Throttle Body Feeback Reading1/1, Error Indication1/1(TBRange), Throttle Body Callibration1/1(TB_Range), TB_Feedbakc Range Conversion1/1(Control Output)
  Foot Pedal Calibration1/2(FP_minVal) -> FP_Input Range Conversion1/3(FP_minVal), ADRC Control1/3(FP_minVal), PID Control1/3(FP_minVal), Foot Pedal Minimum Reading1/1, TB_Feedbakc Range Conversion1/5(FP_minVal)
  No Control1/1(Propotional) -> Operation Selector1/1(Propotional)
  Constant/1 -> Switch/1
  Throttle Body Callibration1/1(TB_maxVal) -> TB Maximum Reading1/1, TB_Feedbakc Range Conversion1/2(TB_maxVal)
  Latching1/2(Button 2) -> [Button_2], Button Control1/2(Bottun 2), If Condition1/2
  Latching1/3(Button 3) -> If Condition1/3, [Button_3], Button Control1/3(Button 3)
  Throttle Body Callibration1/2(TB_minVal) -> TB Minimum Reading1/1, TB_Feedbakc Range Conversion1/3(TB_minVal)
  Foot Pedal Calibration1/1(FP_maxVal) -> FP_Input Range Conversion1/2(FP_maxVal), PID Control1/2(FP_maxVal), ADRC Control1/2(FP_maxVal), Foot Pedal Maximum Reading1/1, TB_Feedbakc Range Conversion1/4(FP_maxVal)
  [Button_3] -> Operation Selector1/6(Switch 3)
  Sum1/1 -> No Control1/1(Error), PID Control1/1(Error), Error Reading1/1, Subsystem3/2(In1)  "Error"
  ADRC Control1/1(ADRC Output) -> Operation Selector1/3(Advanced Control)
  Subsystem3/1(Percentage Error) -> TB New Range Reading3/1  "Percentage Error"
  [Propotional] -> No Control1/Action
  Latching1/1(Button 1) -> [Button_1], Button Control1/1(Button 1), If Condition1/1
  PID Control1/1(PID Output) -> Operation Selector1/2(PID Output), PID Output Reading1/1
  If Condition1/1 -> [Propotional]
  [Button_1] -> Operation Selector1/4(Switch 1)
  [Advance_Control] -> ADRC Control1/Action
  Analog Signal1/1(Out1) -> Throttle Body Feeback Reading (Unused)1/1
  Operation Selector1/1(Control Output) -> FP_Input Range Conversion1/1(Control Output)
  If Condition1/2 -> [PID_Control]
  [Button_2] -> Operation Selector1/5(Switch 2)
  [PID_Control] -> PID Control1/Action
